simulink model "Junctions2_tmp"  (Simulink 8.3)
settings: Solver=ode45  StartTime=0.0  StopTime=10.0  RelTol=1e-3
settings Model: Creator=scaife  LastModifiedBy=bourbouh  CovSFcnEnable=on  ExtModeAutoUpdateStatusClock=off
settings DataIOCC: SignalLoggingName=sigsOut
settings DebuggingCC: SaveWithParameterizedLinksMsg=none  SignalResolutionControl=TryResolveAllWithWarning  SolverPrmCheckMsg=none  MultiTaskDSMMsg=warning  MultiTaskCondExecSysMsg=none  FrameProcessingCompatibilityMsg=error  StateNameClashWarn=none
settings HardwareCC: TargetUnknown=on
settings SFSimCC: SimParseCustomCode=off
settings GRTTargetCC: GeneratePreprocessorConditionals=Use local settings

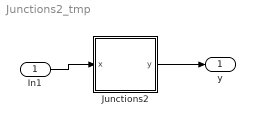
== system Junctions2_tmp ==
  In1 : Inport
  Junctions2 : Stateflow chart  TreatAsAtomicUnit=on
      settings: PermitHierarchicalResolution=ParametersOnly
  y : Outport
  wires:
  In1/1 -> Junctions2/1(x)
  Junctions2/1(y) -> y/1

== stateflow chart Junctions2 ==
  state A
  state B
  state C
  state D
  (default) -> A
  D -> A : [x==0]
  A -> (junction 9) : [x>0]{y++}
  (junction 9) -> (junction 10) [order 1] : [x>=2]{y+=100}
  (junction 10) -> D [order 1] : [x>=4]
      | {y+=10000}
  (junction 9) -> B [order 2] : [x<2]{y+=10}
  (junction 10) -> C [order 2] : [x<4]{y+=1000}
  C -> D : [x==0]
  B -> C : [x==0]
  data: x input int32; y output int32 =11111
